simulink model "Cascaded_PI_Zero_Ref_Test"  (R2023a)
settings: Solver=VariableStepAuto  StartTime=0.0  StopTime=10.0  RelTol=1e-3
values from neighbouring files (symbols this model uses):
  b = 0.490    (= 0.49)    [Cascaded_PI_Step.m]    (also in Cascaded_PI_Zero_Ref.m; Gain_Scheduled_PI_Step.m; Gain_Scheduled_PI_Zero_Ref.m; Inner_Loop_Relay_Feedback.m)
  Clda = 0.65    [Cascaded_PI_Step.m]    (also in Cascaded_PI_Zero_Ref.m; Gain_Scheduled_PI_Step.m; Gain_Scheduled_PI_Zero_Ref.m; Inner_Loop_Relay_Feedback.m)
  Clo = 1.108    [Cascaded_PI_Step.m]    (also in Cascaded_PI_Zero_Ref.m; Gain_Scheduled_PI_Step.m; Gain_Scheduled_PI_Zero_Ref.m; Inner_Loop_Relay_Feedback.m)
  Clp = -1.5    [Cascaded_PI_Step.m]    (also in Cascaded_PI_Zero_Ref.m = -11.5; Gain_Scheduled_PI_Step.m = -11.5; Gain_Scheduled_PI_Zero_Ref.m = -11.5; Inner_Loop_Relay_Feedback.m = -11.5)
  Kc1 = 0.23    [Cascaded_PI_Step.m]    (also in Cascaded_PI_Zero_Ref.m)
  Kc2 = 7.67    [Cascaded_PI_Step.m]    (also in Cascaded_PI_Zero_Ref.m; Gain_Scheduled_PI_Step.m; Gain_Scheduled_PI_Zero_Ref.m; Tethered_Wind_Tunnel.m)
  phi_des = 30    [Cascaded_PI_Step.m]    (also in Cascaded_PI_Zero_Ref.m = 0; Gain_Scheduled_PI_Step.m; Gain_Scheduled_PI_Zero_Ref.m = 0; Outer_Loop_Relay_Feedback.m = 20)
  rho = 1.204    [Cascaded_PI_Step.m]    (also in Cascaded_PI_Zero_Ref.m; Gain_Scheduled_PI_Step.m; Gain_Scheduled_PI_Zero_Ref.m; Inner_Loop_Relay_Feedback.m)
  S = 0.44    [Cascaded_PI_Step.m]    (also in Cascaded_PI_Zero_Ref.m; Gain_Scheduled_PI_Step.m; Gain_Scheduled_PI_Zero_Ref.m; Inner_Loop_Relay_Feedback.m)
  tau1 = 0.146    [Cascaded_PI_Step.m]    (also in Cascaded_PI_Zero_Ref.m)
  tau2 = 24.12    [Cascaded_PI_Step.m]    (also in Cascaded_PI_Zero_Ref.m; Gain_Scheduled_PI_Step.m; Gain_Scheduled_PI_Zero_Ref.m; Tethered_Wind_Tunnel.m)
  Va = 15    [Cascaded_PI_Step.m]    (also in Cascaded_PI_Zero_Ref.m; Gain_Scheduled_PI_Step.m; Gain_Scheduled_PI_Zero_Ref.m; Inner_Loop_Relay_Feedback.m)
libraries: slpidlib x2
settings Model: Creator=brend  LastModifiedBy=brend

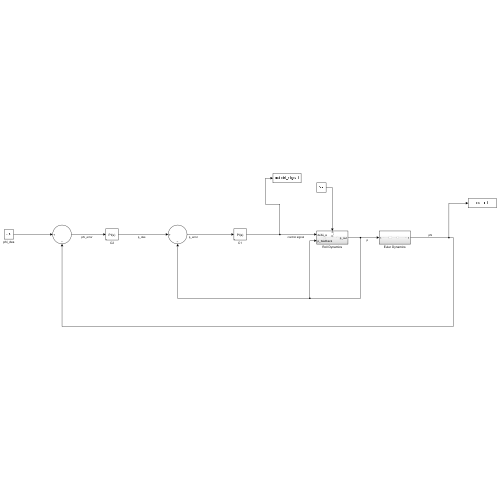
[thumbnail: Simulink's stored preview of the top-level diagram]
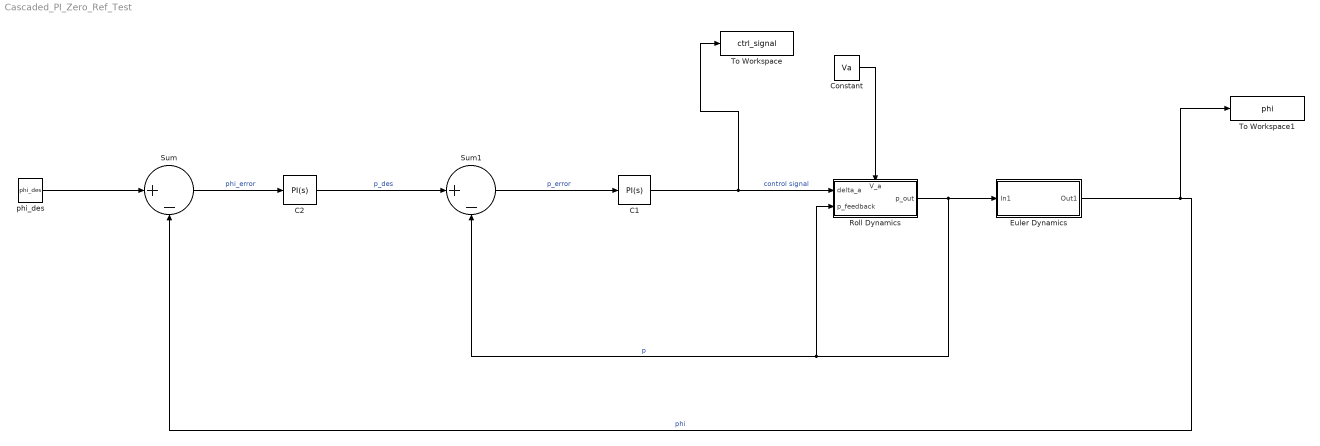
== system Cascaded_PI_Zero_Ref_Test ==
  C1 : slpidlib/PID Controller  Controller=PI  Form=Parallel  TimeDomain=Continuous-time  UseExternalTs=off  SampleTime=-1  IntegratorMethod=Forward Euler  FilterMethod=Forward Euler  ControllerParametersSource=internal  P=Kc1  I=tau1  UseKiTs=off  D=0  N=100  UseFilter=on  TunerSelectOption=Transfer Function Based (PID Tuner App)  InitialConditionSource=internal  InitialConditionForIntegrator=0  InitialConditionForFilter=0  DifferentiatorICPrevScaledInput=0  ExternalReset=none  TrackingMode=off  Kt=1  LimitOutput=off  SatLimitsSource=internal  UpperSaturationLimit=inf  LowerSaturationLimit=-inf  LinearizeAsGain=on  AntiWindupMode=none  Kb=1  LimitIntegrator=off  UpperIntegratorSaturationLimit=inf  LowerIntegratorSaturationLimit=-inf  POutMin=[]  POutMax=[]  IOutMin=[]  IOutMax=[]  DOutMin=[]  DOutMax=[]  NOutMin=[]  NOutMax=[]  SumOutMin=[]  SumOutMax=[]  SaturationOutMin=[]  SaturationOutMax=[]  PParamMin=[]  PParamMax=[]  IParamMin=[]  IParamMax=[]  DParamMin=[]  DParamMax=[]  NParamMin=[]  NParamMax=[]  KbParamMin=[]  KbParamMax=[]  KtParamMin=[]  KtParamMax=[]  KbOutMin=[]  KbOutMax=[]  KtOutMin=[]  KtOutMax=[]  IntegratorOutMin=[]  IntegratorOutMax=[]  FilterOutMin=[]  FilterOutMax=[]  SumI1OutMin=[]  SumI1OutMax=[]  SumI2OutMin=[]  SumI2OutMax=[]  SumI3OutMin=[]  SumI3OutMax=[]  SumI4OutMin=[]  SumI4OutMax=[]  SumDOutMin=[]  SumDOutMax=[]  DifferentiatorOutMin=[]  DifferentiatorOutMax=[]  FilterDiffOutCoefMin=[]  FilterDiffOutCoefMax=[]  ReciprocalOutMin=[]  ReciprocalOutMax=[]  SumDenOutMin=[]  SumDenOutMax=[]  SumNumOutMin=[]  SumNumOutMax=[]  DivideOutMin=[]  DivideOutMax=[]  UdiffTsProdOutMin=[]  UdiffTsProdOutMax=[]  NTsProdOutMin=[]  NTsProdOutMax=[]  UintegralTsProdOutMin=[]  UintegralTsProdOutMax=[]  UngainTsProdOutMin=[]  UngainTsProdOutMax=[]  ClampingZeroOutDataTypeStr=Inherit: Inherit via back propagation  ClampingZeroOutMin=[]  ClampingZeroOutMax=[]  FilterDenConstantOutDataTypeStr=Inherit: Inherit via back propagation  FilterDenConstantOutMin=[]  FilterDenConstantOutMax=[]  PCopyOutDataTypeStr=Inherit: Inherit via back propagation  PCopyOutMin=[]  PCopyOutMax=[]  NCopyOutDataTypeStr=Inherit: Inherit via back propagation  NCopyOutMin=[]  NCopyOutMax=[]  IntegratorContinuousStateAttributes=''  IntegratorStateMustResolveToSignalObject=off  IntegratorRTWStateStorageClass=Auto  FilterContinuousStateAttributes=''  FilterStateMustResolveToSignalObject=off  FilterRTWStateStorageClass=Auto  ParallelPVariant=InternalParameters  IdealPVariant=Disabled  IVariant=InternalParameters  DVariant=Disabled  IntegratorVariant=Continuous  SatVariant=Disabled  AWVariant=Passthrough  PCopyVariant=Disabled  TRVariant=Disabled  FdbkBlocksVariant=Forward  IdealPFdbkVariant=Disabled  SatFdbkVariant=Disabled  DerivativeFilterVariant=Disabled  NVariant=Disabled  NCopyVariant=Disabled_SignalSpec  FilterICVariant=Disabled  IntegratorICVariant=InternalICs  ExternalResetVariant=Disabled  TRSumVariant=Passthrough  SumFdbkVariant=Disabled  SumVariant=Sum_PI  TsampFilterVariant=InternalTs  TsampNgainVariant=Passthrough  TsampIntegralVariant=Disabled_SignalSpec  ExternalSaturationOutDataTypeStr=Inherit: Same as second input
  C2 : slpidlib/PID Controller  Controller=PI  Form=Parallel  TimeDomain=Continuous-time  UseExternalTs=off  SampleTime=-1  IntegratorMethod=Forward Euler  FilterMethod=Forward Euler  ControllerParametersSource=internal  P=Kc2  I=tau2  UseKiTs=off  D=0  N=100  UseFilter=on  TunerSelectOption=Transfer Function Based (PID Tuner App)  InitialConditionSource=internal  InitialConditionForIntegrator=0  InitialConditionForFilter=0  DifferentiatorICPrevScaledInput=0  ExternalReset=none  TrackingMode=off  Kt=1  LimitOutput=off  SatLimitsSource=internal  UpperSaturationLimit=inf  LowerSaturationLimit=-inf  LinearizeAsGain=on  AntiWindupMode=none  Kb=1  LimitIntegrator=off  UpperIntegratorSaturationLimit=inf  LowerIntegratorSaturationLimit=-inf  POutMin=[]  POutMax=[]  IOutMin=[]  IOutMax=[]  DOutMin=[]  DOutMax=[]  NOutMin=[]  NOutMax=[]  SumOutMin=[]  SumOutMax=[]  SaturationOutMin=[]  SaturationOutMax=[]  PParamMin=[]  PParamMax=[]  IParamMin=[]  IParamMax=[]  DParamMin=[]  DParamMax=[]  NParamMin=[]  NParamMax=[]  KbParamMin=[]  KbParamMax=[]  KtParamMin=[]  KtParamMax=[]  KbOutMin=[]  KbOutMax=[]  KtOutMin=[]  KtOutMax=[]  IntegratorOutMin=[]  IntegratorOutMax=[]  FilterOutMin=[]  FilterOutMax=[]  SumI1OutMin=[]  SumI1OutMax=[]  SumI2OutMin=[]  SumI2OutMax=[]  SumI3OutMin=[]  SumI3OutMax=[]  SumI4OutMin=[]  SumI4OutMax=[]  SumDOutMin=[]  SumDOutMax=[]  DifferentiatorOutMin=[]  DifferentiatorOutMax=[]  FilterDiffOutCoefMin=[]  FilterDiffOutCoefMax=[]  ReciprocalOutMin=[]  ReciprocalOutMax=[]  SumDenOutMin=[]  SumDenOutMax=[]  SumNumOutMin=[]  SumNumOutMax=[]  DivideOutMin=[]  DivideOutMax=[]  UdiffTsProdOutMin=[]  UdiffTsProdOutMax=[]  NTsProdOutMin=[]  NTsProdOutMax=[]  UintegralTsProdOutMin=[]  UintegralTsProdOutMax=[]  UngainTsProdOutMin=[]  UngainTsProdOutMax=[]  ClampingZeroOutDataTypeStr=Inherit: Inherit via back propagation  ClampingZeroOutMin=[]  ClampingZeroOutMax=[]  FilterDenConstantOutDataTypeStr=Inherit: Inherit via back propagation  FilterDenConstantOutMin=[]  FilterDenConstantOutMax=[]  PCopyOutDataTypeStr=Inherit: Inherit via back propagation  PCopyOutMin=[]  PCopyOutMax=[]  NCopyOutDataTypeStr=Inherit: Inherit via back propagation  NCopyOutMin=[]  NCopyOutMax=[]  IntegratorContinuousStateAttributes=''  IntegratorStateMustResolveToSignalObject=off  IntegratorRTWStateStorageClass=Auto  FilterContinuousStateAttributes=''  FilterStateMustResolveToSignalObject=off  FilterRTWStateStorageClass=Auto  ParallelPVariant=InternalParameters  IdealPVariant=Disabled  IVariant=InternalParameters  DVariant=Disabled  IntegratorVariant=Continuous  SatVariant=Disabled  AWVariant=Passthrough  PCopyVariant=Disabled  TRVariant=Disabled  FdbkBlocksVariant=Forward  IdealPFdbkVariant=Disabled  SatFdbkVariant=Disabled  DerivativeFilterVariant=Disabled  NVariant=Disabled  NCopyVariant=Disabled_SignalSpec  FilterICVariant=Disabled  IntegratorICVariant=InternalICs  ExternalResetVariant=Disabled  TRSumVariant=Passthrough  SumFdbkVariant=Disabled  SumVariant=Sum_PI  TsampFilterVariant=InternalTs  TsampNgainVariant=Passthrough  TsampIntegralVariant=Disabled_SignalSpec  ExternalSaturationOutDataTypeStr=Inherit: Same as second input
  Constant : Constant  Value=Va
  Euler Dynamics : Subsystem
  Roll Dynamics : Subsystem
      settings: PortSchema="{\"entries\":[{\"content\":{\"sides\":[{\"content\":{\"connectorIds\":[\"In1\",\"In2\"]},\"type\":\"ConnectorPlacement.EquallySpacedRectSide\",\"uuid\":\"0ac85a74-38c1-4d65-b1c0-9ca36de2cddb\"},{\"content\":{\"connectorIds\":[\"Out1\"],\"side\":\"RIGHT\"},\"type\":\"ConnectorPlacement.EquallySpacedRectSide\",\"uuid\":\"84e324c4-b4ec-429b-b00b-3022433bb281\"},{\"content\":{\"connectorIds\":[\"In3\"],\"side\":\"TOP\"},\"type\":\"ConnectorPlacement.EquallySpacedRectSide\",\"uuid\":\"b4486eb0-6e0f-4f77-80f0-5dbcf5ffe993\"}]},\"type\":\"ConnectorPlacement.EquallySpacedConnector\",\"uuid\":\"7fd31f13-990e-44ec-9889-e700ea070706\"}],\"packageUris\":[\"http://schema.mathworks.com/mf0/Connector/R2020b\"],\"version\":\"1.0\"}"
  Sum : Sum  Inputs=|+-
  Sum1 : Sum  Inputs=|+-
  To Workspace : ToWorkspace  VariableName=ctrl_signal  SaveFormat=Timeseries  SampleTime=-1
  To Workspace1 : ToWorkspace  VariableName=phi  SaveFormat=Timeseries  SampleTime=-1
  phi_des : Constant  Value=phi_des
  wires:
  Euler Dynamics/1(Out1) -> To Workspace1/1, Sum/2  "phi"
  Sum1/1 -> C1/1  "p_error"
  C2/1 -> Sum1/1  "p_des"
  phi_des/1 -> Sum/1
  C1/1 -> To Workspace/1, Roll Dynamics/1(delta_a)  "control signal"
  Roll Dynamics/1(p_out) -> Euler Dynamics/1(In1), Sum1/2, Roll Dynamics/2(p_feedback)  "p"
  Constant/1 -> Roll Dynamics/3(V_a)
  Sum/1 -> C2/1  "phi_error"

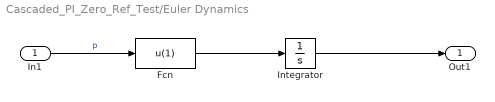
== system Cascaded_PI_Zero_Ref_Test/Euler Dynamics ==
  In1 : Inport
  Fcn : Fcn  Expr=u(1)
  Integrator : Integrator
  Out1 : Outport
  wires:
  In1/1 -> Fcn/1  "p"
  Integrator/1 -> Out1/1
  Fcn/1 -> Integrator/1

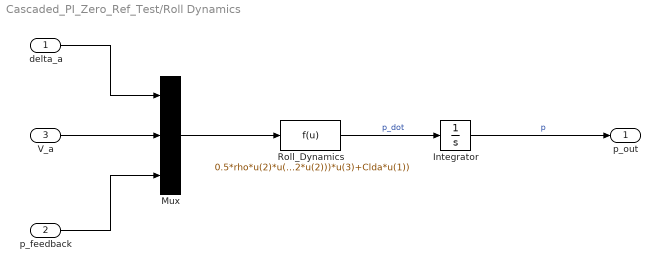
== system Cascaded_PI_Zero_Ref_Test/Roll Dynamics ==
  delta_a : Inport
  p_feedback : Inport  Port=2
  V_a : Inport  Port=3
  Integrator : Integrator
  Mux : Mux  Inputs=3
  Roll_Dynamics : Fcn  Expr=0.5*rho*u(2)*u(2)*S*b*(Clo + Clp*(b/(2*u(2)))*u(3)+Clda*u(1))
  p_out : Outport
  wires:
  delta_a/1 -> Mux/1
  Mux/1 -> Roll_Dynamics/1
  Integrator/1 -> p_out/1  "p"
  V_a/1 -> Mux/2
  p_feedback/1 -> Mux/3
  Roll_Dynamics/1 -> Integrator/1  "p_dot"
